simulink model "Traffic_Light_cs"  (R2019b)
settings: Solver=ode5  StartTime=0.0  StopTime=200  FixedStep=1/1000  RelTol=1e-3
PreLoadFcn:
  | mbxruntime.callbacks.PreLoadFcn(bdroot);
PostLoadFcn:
  | mbxruntime.callbacks.PostLoadFcn(bdroot);
InitFcn:
  | mbxruntime.callbacks.InitFcn(bdroot);
StartFcn:
  | mbxruntime.callbacks.StartFcn(bdroot);
StopFcn:
  | mbxruntime.callbacks.StopFcn(bdroot);
model workspace (MAT data in the model file):
  mbox_table : object (value not decoded)
  model_closed = 0
  sim_status = 0
values from neighbouring files (symbols this model uses):
  load_x1 = [-876.8956 -876.745665143 -876.595730285 -876.445795428 -876.29586057 -876.145925713 -875.995990855 -875.846055998 -875.69612114 -875.546186283 -875.396251425 -875.246316568 ... (5741 elements, 5741x1)]    [Data_ckx.mat]    (also in Load.mat)
  load_y1 = [537.3585 537.354079761 537.349659522 537.345239282 537.340819043 537.336398804 537.331978565 537.327558325 537.323138086 537.318717847 537.314297608 537.309877368 ... (5741 elements, 5741x1)]    [Data_ckx.mat]    (also in Load.mat)
  load_z1 = [0 0 0 0 0 0 0 0 0 0 0 0 ... (5741 elements, 5741x1)]    [Data_ckx.mat]    (also in Load.mat)
  q_pass = [0 0 0 37.0489514481 49.8894252687 51.0913174965 61.791576133 65.4762304223 75.669686677 80.4628164105 88.6197377629 94.2384891559 ... (437675 elements, 87535x5)]    [Data_ckx.mat]
  q_stop = [0 0 0 15.0544571491 15.7911831418 16.0935138936 18.6666396431 19.4721381181 21.7098800606 22.5642135149 25.0883481215 26.1253405703 ... (437675 elements, 87535x5)]    [Data_ckx.mat]
  s = roadinf.s    [Constraint_T_V.m]    (also in Light_Distinguish_old.m = 75:-0.7:75-84*0.7)
undefined symbols (not defined in the file or in its folder): InitImageOutputDir, mbxruntime, sigbuilder_block, tabledata
libraries: simulink x10, PreScanSimulinkLibrary x8, simulink_extras x4, autolibshared x1, fuzblock x1
(part 4 of 5)

== system Traffic_Light_cs/CAR_Main/Decision/Function-Call Subsystem/Subsystem ==
  Dis : Inport
  "CameraSensor " : Inport  Port=2
  traffic_state : Inport  Port=3
  TrafficLight_ID_Main : Inport  Port=4
  function : TriggerPort  TriggerType=function-call  VariantControl=Variant
  Bus Selector1 : BusSelector  OutputSignals=ID1,ID2,ID3
  CameraSensor_0919_100_CM_Demux : Subsystem  Tag=demux/Camera/Color  Commented=on  mask{SensorName=CameraSensor_0919_100, hres=1920, vres=1800}
      mask prompts: SensorName "Sensor Name"; hres "Horizontal Resolution"; vres "Vertical Resolution"
      mask Help: eval('openHelp(457)')
      mask Display:
      | fprintf('MONO CAMERA:\n Color\n %s \n %d x %d px',SensorName,hres,vres)
      | port_label('output',1,'R')
      | port_label('output',2,'G')
      | port_label('output',3,'B')
  Constant : Constant  Commented=on  Value=14
  Delay : Stateflow chart  TreatAsAtomicUnit=on
  From : From  Commented=on  GotoTag=R_Ori
  From1 : From  Commented=on  GotoTag=G_Ori
  From2 : From  Commented=on  GotoTag=B_Ori
  Goto : Goto  Commented=on  GotoTag=R_Ori
  Goto1 : Goto  Commented=on  GotoTag=G_Ori
  Goto2 : Goto  Commented=on  GotoTag=B_Ori
  MATLAB Function : MATLAB Function  Commented=on  TreatAsAtomicUnit=on
  MATLAB Function1 : MATLAB Function  TreatAsAtomicUnit=on
  Multiport Switch1 : MultiPortSwitch  DiagnosticForDefault=None
  Product : Product  Commented=on
  Sqrt : Sqrt  Commented=on  SaturateOnIntegerOverflow=on
  Sum : Sum  Commented=on  Inputs=|-+
  Light_State_0919_100 : Outport  VectorParamsAs1DForOutWhenUnconnected=off
  wires:
  Delay/1(Light_State_End) -> Light_State_0919_100/1
  Sqrt/1 -> MATLAB Function/1(Dis)
  Sum/1 -> Sqrt/1
  Constant/1 -> Sum/1
  Product/1 -> Sum/2
  Dis/1 -> MATLAB Function1/1(u), Product/2, Product/1
  From2/1 -> MATLAB Function/4(B_Ori)
  CameraSensor_0919_100_CM_Demux/3(B) -> Goto2/1
  MATLAB Function/1(Light_State) -> ?  "Light_State_0919_100"
  CameraSensor_0919_100_CM_Demux/2(G) -> Goto1/1
  CameraSensor_0919_100_CM_Demux/1(R) -> Goto/1
  "CameraSensor "/1 -> CameraSensor_0919_100_CM_Demux/1(In1)
  From1/1 -> MATLAB Function/3(G_Ori)
  From/1 -> MATLAB Function/2(R_Ori)
  Multiport Switch1/1 -> MATLAB Function1/2(data)
  traffic_state/1 -> Bus Selector1/1
  Bus Selector1/1 -> Multiport Switch1/2  "<ID1>"
  Bus Selector1/2 -> Multiport Switch1/3  "<ID2>"
  Bus Selector1/3 -> Multiport Switch1/4  "<ID3>"
  TrafficLight_ID_Main/1 -> Multiport Switch1/1
  MATLAB Function1/1(y) -> Delay/1(Light_State_0919_100)

== system Traffic_Light_cs/CAR_Main/Dynamics_Simple/Chassis/Bicycle_model_[XYZ] ==
  DeltaWheel_[rad] : Inport
  zFront_[m]_dzFront_[ms-1] : Inport  Port=2  PortDimensions=2
  zRear_[m]_dzRear_[ms-1] : Inport  Port=3  PortDimensions=2
  |vx|_[ms-1] : Inport  Port=4
  Fy_rear_[N] : Inport  Port=5
  Fy_front_[N] : Inport  Port=6
  Demux : Demux  Outputs=2
  Demux1 : Demux  Outputs=2
  Fyi --> Fy / Mz : Subsystem
  Y & Yaw_Motion : Subsystem
  "Z, Pitch_Motion & Roll_Motion" : Subsystem
  |vx|_[ms-1]1 : Outport  VectorParamsAs1DForOutWhenUnconnected=off
  vy_[ms-1] : Outport  Port=2  VectorParamsAs1DForOutWhenUnconnected=off
  vz_[ms-1] : Outport  Port=3  VectorParamsAs1DForOutWhenUnconnected=off
  RollAngle_[rad] : Outport  Port=4  VectorParamsAs1DForOutWhenUnconnected=off
  RollRate_[rads-1] : Outport  Port=5  VectorParamsAs1DForOutWhenUnconnected=off
  YawAngle_[rads-1] : Outport  Port=6  VectorParamsAs1DForOutWhenUnconnected=off
  PitchAngle_[rad] : Outport  Port=7  VectorParamsAs1DForOutWhenUnconnected=off
  YawAngle_[rad] : Outport  Port=8  VectorParamsAs1DForOutWhenUnconnected=off
  ay_[ms-2] : Outport  Port=9  VectorParamsAs1DForOutWhenUnconnected=off
  wires:
  "Z, Pitch_Motion & Roll_Motion"/1(pitchAngle_[rad]) -> PitchAngle_[rad]/1  "PitchAngle_[rad]"
  Y & Yaw_Motion/4(dYawAngle_[rads-1]) -> [dYaw], YawAngle_[rads-1]/1  "dYawAngle_[rads-1]"
  [vx] -> "Z, Pitch_Motion & Roll_Motion"/1(vx)
  [dYaw] -> "Z, Pitch_Motion & Roll_Motion"/2(dYaw)
  "Z, Pitch_Motion & Roll_Motion"/4(RollRate_[rads-1]) -> RollRate_[rads-1]/1  "RollRate_[rads-1]"
  "Z, Pitch_Motion & Roll_Motion"/3(RollAngle_[rad]) -> RollAngle_[rad]/1  "RollAngle_[rad]"
  [ay] -> "Z, Pitch_Motion & Roll_Motion"/4(ay)
  Y & Yaw_Motion/3(ay_[ms-2]) -> ay_[ms-2]/1, [ay]  "ay_[ms-2]"
  |vx|_[ms-1]/1 -> Y & Yaw_Motion/1(|vx|_[ms-1])
  Fy_rear_[N]/1 -> Fyi --> Fy / Mz/3(Fy_r_[N])
  Fy_front_[N]/1 -> Fyi --> Fy / Mz/2(Fy_f_[N])
  DeltaWheel_[rad]/1 -> Fyi --> Fy / Mz/1(DeltaWheel_[rad])
  "Z, Pitch_Motion & Roll_Motion"/2(vz_[ms-1]) -> vz_[ms-1]/1  "vz_[ms-1]"
  zFront_[m]_dzFront_[ms-1]/1 -> Demux/1
  zRear_[m]_dzRear_[ms-1]/1 -> Demux1/1
  Demux1/2 -> "Z, Pitch_Motion & Roll_Motion"/8(dzRear_[ms-1])
  Demux1/1 -> "Z, Pitch_Motion & Roll_Motion"/7(zRear_[m])
  Demux/2 -> "Z, Pitch_Motion & Roll_Motion"/6(dzFront_[ms-1])
  Demux/1 -> "Z, Pitch_Motion & Roll_Motion"/5(zFront_[m])
  [ax] -> "Z, Pitch_Motion & Roll_Motion"/3(ax)
  Y & Yaw_Motion/5(YawAngle_[rad]) -> YawAngle_[rad]/1  "YawAngle_[rad]"
  Y & Yaw_Motion/2(vy_[ms-1]) -> vy_[ms-1]/1  "vy_[ms-1]"
  Y & Yaw_Motion/1(|vx|_[ms-1]1) -> |vx|_[ms-1]1/1  "|vx|_[ms-1]"
  Fyi --> Fy / Mz/2(Mz_[Nm]) -> Y & Yaw_Motion/3(Mz_[Nm])  "Mz_[Nm]"
  Fyi --> Fy / Mz/1(Fy_[N]) -> Y & Yaw_Motion/2(Fy_[N])  "Fy_[N]"

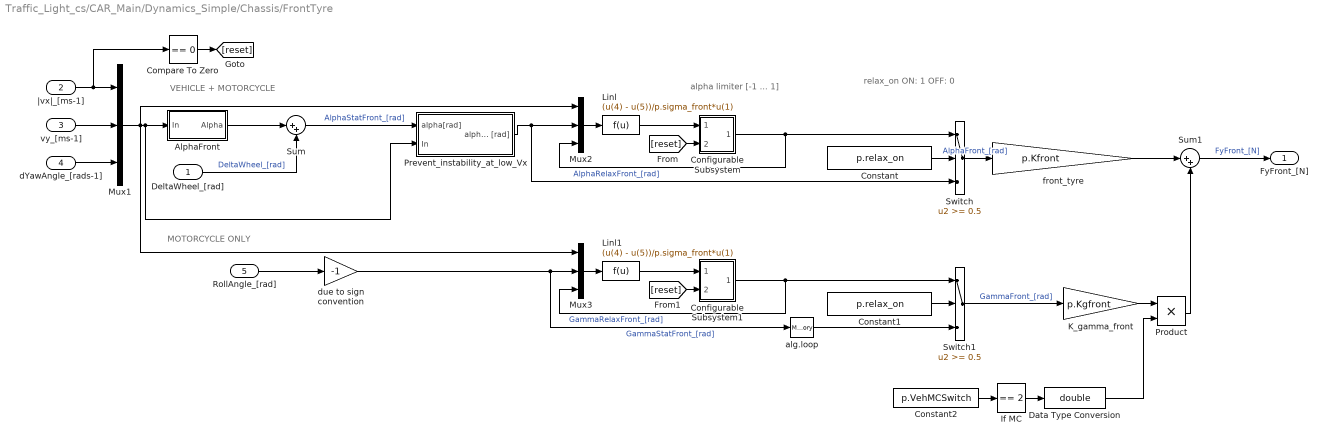
== system Traffic_Light_cs/CAR_Main/Dynamics_Simple/Chassis/FrontTyre ==
  note: VEHICLE + MOTORCYCLE
  note: MOTORCYCLE ONLY
  note: relax_on
      | ON: 1
      | OFF: 0
  note: alpha limiter
      | [-1 ... 1]
  DeltaWheel_[rad] : Inport
  |vx|_[ms-1] : Inport  Port=2
  vy_[ms-1] : Inport  Port=3
  dYawAngle_[rads-1] : Inport  Port=4
  RollAngle_[rad] : Inport  Port=5
  AlphaFront : Subsystem
  Compare To Zero : simulink/Logic and Bit Operations/Compare To Zero  relop===  OutDataTypeStr=boolean  ZeroCross=off
  Configurable Subsystem : Subsystem  BlockChoice=Integrator  mask{ComputationMode=ComputationMode}
      mask prompts: ComputationMode "Computation mode:"
      mask init:
      | SetComputationMode(gcb,ComputationMode);
      settings: AttributesFormatString=%<BlockChoice>  OpenFcn=BringToFront(gcb);  MemberBlocks=Discrete-Time Integrator,Integrator
      settings: TemplateBlock=|
      | PreScanSimulinkLibrary/Configurable Subsystems/integral with reset and limits
      | for slip angle/Configurable
      | Subsystem
  Configurable Subsystem1 : Subsystem  BlockChoice=Integrator  mask{ComputationMode=ComputationMode}
      mask prompts: ComputationMode "Computation mode:"
      mask init:
      | SetComputationMode(gcb,ComputationMode);
      settings: AttributesFormatString=%<BlockChoice>  OpenFcn=BringToFront(gcb);  MemberBlocks=Discrete-Time Integrator,Integrator
      settings: TemplateBlock=|
      | PreScanSimulinkLibrary/Configurable Subsystems/integral with reset/Configurable
      | Subsystem
  Constant : Constant  Value=p.relax_on
  Constant1 : Constant  Value=p.relax_on
  Constant2 : Constant  Value=p.VehMCSwitch
  Data Type Conversion : DataTypeConversion  OutDataTypeStr=double
  If MC : simulink/Logic and Bit Operations/Compare To Constant  relop===  const=2  OutDataTypeStr=uint8  ZeroCross=off
  K_gamma_front : Gain  Gain=p.Kgfront
  Linl : Fcn  Expr=(u(4) - u(5))/p.sigma_front*u(1)
  Linl1 : Fcn  Expr=(u(4) - u(5))/p.sigma_front*u(1)
  Mux1 : Mux  Inputs=3
  Mux2 : Mux  Inputs={3,1,1}
  Mux3 : Mux  Inputs={3,1,1}
  Prevent_instability_at_low_Vx : Subsystem
  Product : Product  RndMeth=Zero
  Sum : Sum  Inputs=|++  SaturateOnIntegerOverflow=on  InputSameDT=on  OutDataTypeStr=Inherit: Same as first input
  Sum1 : Sum  Inputs=|++
  Switch : Switch  Threshold=0.5  SaturateOnIntegerOverflow=on  InputSameDT=on
  Switch1 : Switch  Threshold=0.5  SaturateOnIntegerOverflow=on  InputSameDT=on
  alg.loop : Memory
  due to sign convention : Gain  Gain=-1  SaturateOnIntegerOverflow=on  OutDataTypeStr=Inherit: Same as input  ParamDataTypeStr=Inherit: Same as input
  front_tyre : Gain  Gain=p.Kfront
  FyFront_[N] : Outport  VectorParamsAs1DForOutWhenUnconnected=off
  wires:
  Switch1/1 -> K_gamma_front/1  "GammaFront_[rad]"
  DeltaWheel_[rad]/1 -> Sum/2  "DeltaWheel_[rad]"
  [reset] -> Configurable Subsystem1/2(In2)
  [reset] -> Configurable Subsystem/2(In2)
  Compare To Zero/1 -> [reset]
  Data Type Conversion/1 -> Product/2
  Product/1 -> Sum1/2
  K_gamma_front/1 -> Product/1
  If MC/1 -> Data Type Conversion/1
  Constant2/1 -> If MC/1
  front_tyre/1 -> Sum1/1
  RollAngle_[rad]/1 -> due to sign convention/1
  due to sign convention/1 -> Mux3/2, alg.loop/1  "GammaStatFront_[rad]"
  Constant1/1 -> Switch1/2
  Mux3/1 -> Linl1/1
  Linl1/1 -> Configurable Subsystem1/1(In1)
  Configurable Subsystem1/1(Out1) -> Switch1/1, Mux3/3  "GammaRelaxFront_[rad]"
  alg.loop/1 -> Switch1/3
  dYawAngle_[rads-1]/1 -> Mux1/3
  vy_[ms-1]/1 -> Mux1/2
  |vx|_[ms-1]/1 -> Compare To Zero/1, Mux1/1
  Mux1/1 -> Mux3/1, Mux2/1, AlphaFront/1(In), Prevent_instability_at_low_Vx/2(In)
  AlphaFront/1(Alpha) -> Sum/1
  Configurable Subsystem/1(Out1) -> Switch/1, Mux2/3  "AlphaRelaxFront_[rad]"
  Linl/1 -> Configurable Subsystem/1(In1)
  Mux2/1 -> Linl/1
  Sum1/1 -> FyFront_[N]/1  "FyFront_[N]"
  Constant/1 -> Switch/2
  Switch/1 -> front_tyre/1  "AlphaFront_[rad]"
  Sum/1 -> Prevent_instability_at_low_Vx/1(alpha[rad])  "AlphaStatFront_[rad]"
  Prevent_instability_at_low_Vx/1(alpha [rad]) -> Switch/3, Mux2/2

== system Traffic_Light_cs/CAR_Main/Dynamics_Simple/Chassis/MuxDynState ==
  note: AnglesVEHICLE
      | wrtGLOB
  note: mode: Dynamics
      | VelVEHICLE
      | wrt VEH
  note: The position inputs are computed by the
      | integrated velocity.
  vx [ms-1] : Inport
  vy [ms-1] : Inport  Port=2
  vz [ms-1] : Inport  Port=3
  R [rad] : Inport  Port=4
  P [rad] : Inport  Port=5
  Y [rad] : Inport  Port=6
  Configurable Subsystem1 : Subsystem  BlockChoice=Integrator  mask{ComputationMode=ComputationMode}
      mask prompts: ComputationMode "Computation mode:"
      mask init:
      | SetComputationMode(gcb,ComputationMode);
      settings: AttributesFormatString=%<BlockChoice>  OpenFcn=BringToFront(gcb);  MemberBlocks=Discrete-Time Integrator,Integrator
      settings: TemplateBlock=|
      | PreScanSimulinkLibrary/Configurable Subsystems/integral/Configurable
      | Subsystem1
  Ground : Ground
  Ground1 : Ground
  Mux : Mux  Inputs=[3 3 3]
  Mux1 : Mux  Inputs=3
  Mux2 : Mux  Inputs=3
  Transformation_BODY2GLOBAL : Subsystem
  mux3 : Mux  Inputs=3
  State : Outport  VectorParamsAs1DForOutWhenUnconnected=off
  wires:
  Configurable Subsystem1/1(Out1) -> Mux/1  "PosVEH wrt  GLOB"
  Mux1/1 -> Transformation_BODY2GLOBAL/1(Vvector_BODY_[m/s])
  Mux/1 -> State/1
  Ground/1 -> mux3/1  "roll"
  mux3/1 -> Transformation_BODY2GLOBAL/2(angles_BODYwrtGLOB_[rad])
  Transformation_BODY2GLOBAL/1(Vvector_GLOBAL_[m/s]) -> Mux/2, Configurable Subsystem1/1(In1)  "VelVEH wrt  GLOB"
  Mux2/1 -> Mux/3
  vx [ms-1]/1 -> Mux1/1
  vy [ms-1]/1 -> Mux1/2
  vz [ms-1]/1 -> Mux1/3
  R [rad]/1 -> Mux2/1
  P [rad]/1 -> Mux2/2
  Y [rad]/1 -> mux3/3, Mux2/3  "yaw"
  Ground1/1 -> mux3/2  "pitch"

== system Traffic_Light_cs/CAR_Main/Dynamics_Simple/Chassis/Power Assisted Steering ==
  note: Reverse steering direction for negative velocities
  note: VEHICLE
  note: MOTORCYCLE
  Vx_[ms-1] : Inport
  Delta_in_[deg] : Inport  Port=2
  Constant : Constant
  Constant1 : Constant  Value=p.VehMCSwitch
  Lookup Table : Lookup  InputValues=[0 35 45 100]  Table=[1 1 0.2 0.2]
  Multiport Switch : MultiPortSwitch  Inputs=2
  Product : Product  Inputs=3  RndMeth=Zero
  Sign : Signum
  Delta_out_[deg] : Outport  VectorParamsAs1DForOutWhenUnconnected=off
  wires:
  Sign/1 -> Product/1
  Product/1 -> Delta_out_[deg]/1
  Multiport Switch/1 -> Product/2
  Lookup Table/1 -> Multiport Switch/2
  Constant/1 -> Multiport Switch/3
  Constant1/1 -> Multiport Switch/1
  Delta_in_[deg]/1 -> Product/3
  Vx_[ms-1]/1 -> Sign/1, Lookup Table/1

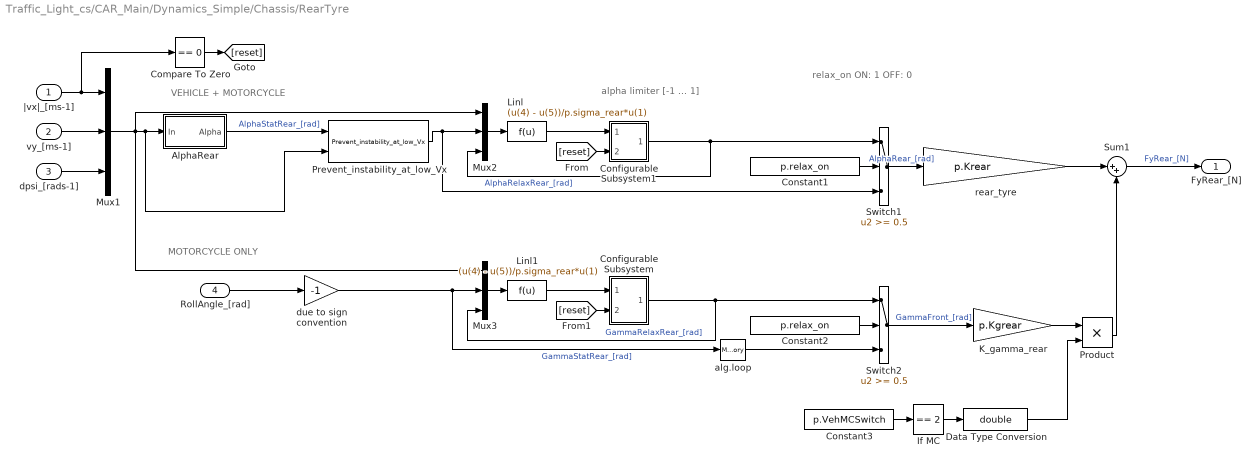
== system Traffic_Light_cs/CAR_Main/Dynamics_Simple/Chassis/RearTyre ==
  note: VEHICLE + MOTORCYCLE
  note: MOTORCYCLE ONLY
  note: relax_on
      | ON: 1
      | OFF: 0
  note: alpha limiter
      | [-1 ... 1]
  |vx|_[ms-1] : Inport
  vy_[ms-1] : Inport  Port=2
  dpsi_[rads-1] : Inport  Port=3
  RollAngle_[rad] : Inport  Port=4
  AlphaRear : Subsystem
  Compare To Zero : simulink/Logic and Bit Operations/Compare To Zero  relop===  OutDataTypeStr=boolean  ZeroCross=off
  Configurable Subsystem : Subsystem  BlockChoice=Integrator  mask{ComputationMode=ComputationMode}
      mask prompts: ComputationMode "Computation mode:"
      mask init:
      | SetComputationMode(gcb,ComputationMode);
      settings: AttributesFormatString=%<BlockChoice>  OpenFcn=BringToFront(gcb);  MemberBlocks=Discrete-Time Integrator,Integrator
      settings: TemplateBlock=|
      | PreScanSimulinkLibrary/Configurable Subsystems/integral with reset/Configurable
      | Subsystem
  Configurable Subsystem1 : Subsystem  BlockChoice=Integrator  mask{ComputationMode=ComputationMode}
      mask prompts: ComputationMode "Computation mode:"
      mask init:
      | SetComputationMode(gcb,ComputationMode);
      settings: AttributesFormatString=%<BlockChoice>  OpenFcn=BringToFront(gcb);  MemberBlocks=Discrete-Time Integrator,Integrator
      settings: TemplateBlock=|
      | PreScanSimulinkLibrary/Configurable Subsystems/integral with reset and limits
      | for slip angle/Configurable
      | Subsystem
  Constant1 : Constant  Value=p.relax_on
  Constant2 : Constant  Value=p.relax_on
  Constant3 : Constant  Value=p.VehMCSwitch
  Data Type Conversion : DataTypeConversion  OutDataTypeStr=double
  If MC : simulink/Logic and Bit Operations/Compare To Constant  relop===  const=2  OutDataTypeStr=uint8  ZeroCross=off
  K_gamma_rear : Gain  Gain=p.Kgrear
  Linl : Fcn  Expr=(u(4) - u(5))/p.sigma_rear*u(1)
  Linl1 : Fcn  Expr=(u(4) - u(5))/p.sigma_rear*u(1)
  Mux1 : Mux  Inputs=3
  Mux2 : Mux  Inputs={3,1,1}
  Mux3 : Mux  Inputs={3,1,1}
  Prevent_instability_at_low_Vx : PreScanSimulinkLibrary/Simple_Vehicle_Dynamics/Chassis/FrontTyre/Prevent_instability_at_low_Vx  SystemSampleTime=-1  Latency=0  AutoFrameSizeCalculation=off
  Product : Product  RndMeth=Zero
  Sum1 : Sum  Inputs=|++
  Switch1 : Switch  Threshold=0.5  SaturateOnIntegerOverflow=on  InputSameDT=on
  Switch2 : Switch  Threshold=0.5  SaturateOnIntegerOverflow=on  InputSameDT=on
  alg.loop : Memory
  due to sign convention : Gain  Gain=-1  SaturateOnIntegerOverflow=on  OutDataTypeStr=Inherit: Same as input  ParamDataTypeStr=Inherit: Same as input
  rear_tyre : Gain  Gain=p.Krear
  FyRear_[N] : Outport  VectorParamsAs1DForOutWhenUnconnected=off
  wires:
  Switch2/1 -> K_gamma_rear/1  "GammaFront_[rad]"
  [reset] -> Configurable Subsystem/2(In2)
  [reset] -> Configurable Subsystem1/2(In2)
  Compare To Zero/1 -> [reset]
  rear_tyre/1 -> Sum1/1
  K_gamma_rear/1 -> Product/1
  Data Type Conversion/1 -> Product/2
  Product/1 -> Sum1/2
  If MC/1 -> Data Type Conversion/1
  Constant3/1 -> If MC/1
  RollAngle_[rad]/1 -> due to sign convention/1
  due to sign convention/1 -> Mux3/2, alg.loop/1  "GammaStatRear_[rad]"
  Constant2/1 -> Switch2/2
  Mux3/1 -> Linl1/1
  Linl1/1 -> Configurable Subsystem/1(In1)
  Configurable Subsystem/1(Out1) -> Switch2/1, Mux3/3  "GammaRelaxRear_[rad]"
  alg.loop/1 -> Switch2/3
  dpsi_[rads-1]/1 -> Mux1/3
  vy_[ms-1]/1 -> Mux1/2
  |vx|_[ms-1]/1 -> Compare To Zero/1, Mux1/1
  Mux1/1 -> Mux3/1, Mux2/1, Prevent_instability_at_low_Vx/2, AlphaRear/1(In)
  Configurable Subsystem1/1(Out1) -> Switch1/1, Mux2/3  "AlphaRelaxRear_[rad]"
  Linl/1 -> Configurable Subsystem1/1(In1)
  Mux2/1 -> Linl/1
  Sum1/1 -> FyRear_[N]/1  "FyRear_[N]"
  Constant1/1 -> Switch1/2
  Switch1/1 -> rear_tyre/1  "AlphaRear_[rad]"
  AlphaRear/1(Alpha) -> Prevent_instability_at_low_Vx/1  "AlphaStatRear_[rad]"
  Prevent_instability_at_low_Vx/1 -> Mux2/2, Switch1/3

== system Traffic_Light_cs/CAR_Main/SELF_Demux/compas converter/cart2compas ==
  Angle [deg] : Inport
  Constant : Constant  Value=90
  Constant1 : Constant  Value=360
  Gain : Gain  Gain=1/360
  Gain1 : Gain  Gain=360
  Gain2 : Gain  Gain=-1
  Rounding Function : Rounding
  Sum : Sum  Inputs=|-+
  Sum1 : Sum  Inputs=-+|
  Sum2 : Sum  Inputs=++|
  heading [deg] : Outport
  wires:
  Gain/1 -> Rounding Function/1
  Rounding Function/1 -> Gain1/1
  Gain1/1 -> Sum/1
  Angle [deg]/1 -> Sum1/2
  Sum/1 -> Gain2/1
  Sum1/1 -> Gain/1, Sum/2
  Constant/1 -> Sum1/1
  Gain2/1 -> Sum2/2
  Constant1/1 -> Sum2/1
  Sum2/1 -> heading [deg]/1

== system Traffic_Light_cs/CAR_Main/pre/Subsystem/Signal Builder ==
  Demux : Demux  Tag=STV Demux  Outputs=6
  FromWs : FromWorkspace  Tag=STV FromWs  VariableName=tuvar  SampleTime=0
      SigBuilderData=|
      | common.afterFinalStr = 'Extrapolate'
      | common.sampleTime = 0
      | dataSet.timeRange = [0 200]
      | dataSet.name = 'Traffic Light GPS Information'
      | sbobj.Groups.Name = 'Traffic Light GPS Information'
      | sbobj.Groups.Signals(1).Name = 'ID==1,X'
      | sbobj.Groups.Signals(1).XData = [0 200]
      | sbobj.Groups.Signals(1).YData = [-610.5 -610.5]
      | sbobj.Groups.Signals(2).Name = 'ID==1,Y'
      | sbobj.Groups.Signals(2).XData = [0 200]
      | sbobj.Groups.Signals(2).YData = [362.27 362.27]
      | sbobj.Groups.Signals(3).Name = 'ID==2,X'
      | sbobj.Groups.Signals(3).XData = [0 200]
      | sbobj.Groups.Signals(3).YData = [-639.42 -639.42]
      | sbobj.Groups.Signals(4).Name = 'ID==2,Y'
      | sbobj.Groups.Signals(4).XData = [0 200]
      | sbobj.Groups.Signals(4).YData = [295.94 295.94]
      | sbobj.Groups.Signals(5).Name = 'ID==3,X'
      | sbobj.Groups.Signals(5).XData = [0 200]
      | sbobj.Groups.Signals(5).YData = [-718.98 -718.98]
      | sbobj.Groups.Signals(6).Name = 'ID==3,Y'
      | sbobj.Groups.Signals(6).XData = [0 200]
      | sbobj.Groups.Signals(6).YData = [201.74 201.74]
      | sbobj.Groups.TimeRange = [0 200]
  ID==1,X : Outport  Tag=STV Outport
  ID==1,Y : Outport  Tag=STV Outport  Port=2  VectorParamsAs1DForOutWhenUnconnected=off
  ID==2,X : Outport  Tag=STV Outport  Port=3  VectorParamsAs1DForOutWhenUnconnected=off
  ID==2,Y : Outport  Tag=STV Outport  Port=4  VectorParamsAs1DForOutWhenUnconnected=off
  ID==3,X : Outport  Tag=STV Outport  Port=5  VectorParamsAs1DForOutWhenUnconnected=off
  ID==3,Y : Outport  Tag=STV Outport  Port=6  VectorParamsAs1DForOutWhenUnconnected=off
  wires:
  Demux/6 -> ID==3,Y/1
  Demux/5 -> ID==3,X/1
  Demux/4 -> ID==2,Y/1
  Demux/3 -> ID==2,X/1
  Demux/2 -> ID==1,Y/1
  Demux/1 -> ID==1,X/1
  FromWs/1 -> Demux/1

== system Traffic_Light_cs/CAR_Ahead/Decision/Function-Call Subsystem/Subsystem/CameraSensor_0919_100_CM_Demux ==
  In1 : Inport
  Selector : Selector  NumberOfDimensions=2  InputPortWidth=3  IndexOptions=Index vector (dialog),Index vector (dialog)  Indices=-1,1:hres  OutputSizes=1,1
  Selector1 : Selector  NumberOfDimensions=2  InputPortWidth=3  IndexOptions=Index vector (dialog),Index vector (dialog)  Indices=-1,hres+1:hres*2  OutputSizes=1,1
  Selector2 : Selector  NumberOfDimensions=2  InputPortWidth=3  IndexOptions=Index vector (dialog),Index vector (dialog)  Indices=-1,hres*2+1:hres*3  OutputSizes=1,1
  R : Outport  VectorParamsAs1DForOutWhenUnconnected=off
  G : Outport  Port=2  VectorParamsAs1DForOutWhenUnconnected=off
  B : Outport  Port=3  VectorParamsAs1DForOutWhenUnconnected=off
  wires:
  Selector2/1 -> B/1
  Selector1/1 -> G/1
  Selector/1 -> R/1
  In1/1 -> Selector2/1, Selector/1, Selector1/1

== system Traffic_Light_cs/CAR_Ahead/Trajectories/Traj2State1/Traj2State2/MuxState ==
  x [m] : Inport
  y [m] : Inport  Port=2
  z [m] : Inport  Port=3
  dx [m/s] : Inport  Port=4
  dy [m/s] : Inport  Port=5
  dz [m/s] : Inport  Port=6
  R [rad] : Inport  Port=7
  P [rad] : Inport  Port=8
  Y [rad] : Inport  Port=9
  Mux : Mux  Inputs=9
  state : Outport
  wires:
  z [m]/1 -> Mux/3
  y [m]/1 -> Mux/2
  x [m]/1 -> Mux/1
  Y [rad]/1 -> Mux/9
  P [rad]/1 -> Mux/8
  R [rad]/1 -> Mux/7
  dz [m/s]/1 -> Mux/6
  dy [m/s]/1 -> Mux/5
  dx [m/s]/1 -> Mux/4
  Mux/1 -> state/1

== system Traffic_Light_cs/CAR_Ahead/Trajectories/Traj2State1/Traj2State2/Traj2MuxState_Ext ==
  Traj : Inport
  Terminator{1..9} (9 alike) : Terminator
  demux : Subsystem
  x [m] : Outport
  y [m] : Outport  Port=2
  z [m] : Outport  Port=3
  dx [m/s] : Outport  Port=4
  dy [m/s] : Outport  Port=5
  dz [m/s] : Outport  Port=6
  R [rad] : Outport  Port=7
  P [rad] : Outport  Port=8
  Y [rad] : Outport  Port=9
  wires:
  demux/9(Y) -> Y [rad]/1
  demux/7(R) -> R [rad]/1
  demux/5(vely) -> dy [m/s]/1
  demux/4(velx) -> dx [m/s]/1
  demux/10(velR) -> Terminator4/1
  demux/11(velP) -> Terminator5/1
  demux/12(velY) -> Terminator1/1
  demux/13(accx) -> Terminator8/1
  demux/14(accy) -> Terminator9/1
  demux/15(accz) -> Terminator7/1
  demux/18(accY) -> Terminator2/1
  demux/16(accR) -> Terminator3/1
  demux/17(accP) -> Terminator6/1
  demux/3(z) -> z [m]/1
  Traj/1 -> demux/1(traj)
  demux/6(velz) -> dz [m/s]/1
  demux/1(x) -> x [m]/1
  demux/2(y) -> y [m]/1
  demux/8(P) -> P [rad]/1

== system Traffic_Light_cs/CAR_Main/Decision/Function-Call Subsystem/Subsystem/CameraSensor_0919_100_CM_Demux ==
  In1 : Inport
  Selector : Selector  NumberOfDimensions=2  InputPortWidth=3  IndexOptions=Index vector (dialog),Index vector (dialog)  Indices=-1,1:hres  OutputSizes=1,1
  Selector1 : Selector  NumberOfDimensions=2  InputPortWidth=3  IndexOptions=Index vector (dialog),Index vector (dialog)  Indices=-1,hres+1:hres*2  OutputSizes=1,1
  Selector2 : Selector  NumberOfDimensions=2  InputPortWidth=3  IndexOptions=Index vector (dialog),Index vector (dialog)  Indices=-1,hres*2+1:hres*3  OutputSizes=1,1
  R : Outport  VectorParamsAs1DForOutWhenUnconnected=off
  G : Outport  Port=2  VectorParamsAs1DForOutWhenUnconnected=off
  B : Outport  Port=3  VectorParamsAs1DForOutWhenUnconnected=off
  wires:
  Selector2/1 -> B/1
  Selector1/1 -> G/1
  Selector/1 -> R/1
  In1/1 -> Selector2/1, Selector/1, Selector1/1

== system Traffic_Light_cs/CAR_Main/Dynamics_Simple/Chassis/Bicycle_model_[XYZ]/Fyi --> Fy // Mz ==
  DeltaWheel_[rad] : Inport
  Fy_f_[N] : Inport  Port=2
  Fy_r_[N] : Inport  Port=3
  Fy : Fcn  Expr=u(2)*cos(u(1)) + u(3)
  Mux1 : Mux  Inputs=3
  Mz : Fcn  Expr=u(2)*p.a*cos(u(1)) - u(3)*p.b
  Fy_[N] : Outport  InitialOutput=0  VectorParamsAs1DForOutWhenUnconnected=off
  Mz_[Nm] : Outport  Port=2  InitialOutput=0  VectorParamsAs1DForOutWhenUnconnected=off
  wires:
  Fy_r_[N]/1 -> Mux1/3
  Fy_f_[N]/1 -> Mux1/2
  Mux1/1 -> Fy/1, Mz/1
  Fy/1 -> Fy_[N]/1
  Mz/1 -> Mz_[Nm]/1
  DeltaWheel_[rad]/1 -> Mux1/1  "DeltaWheel_[rad]"

== system Traffic_Light_cs/CAR_Main/Dynamics_Simple/Chassis/Bicycle_model_[XYZ]/Y & Yaw_Motion ==
  |vx|_[ms-1] : Inport
  Fy_[N] : Inport  Port=2
  Mz_[Nm] : Inport  Port=3
  Compare To Zero : simulink/Logic and Bit Operations/Compare To Zero  relop===  OutDataTypeStr=boolean  ZeroCross=off
  Configurable Subsystem : Subsystem  BlockChoice=Integrator  mask{ComputationMode=ComputationMode}
      mask prompts: ComputationMode "Computation mode:"
      mask init:
      | SetComputationMode(gcb,ComputationMode);
      settings: AttributesFormatString=%<BlockChoice>  OpenFcn=BringToFront(gcb);  MemberBlocks=Discrete-Time Integrator,Integrator
      settings: TemplateBlock=|
      | PreScanSimulinkLibrary/Configurable Subsystems/integral with reset/Configurable
      | Subsystem
  Configurable Subsystem1 : Subsystem  BlockChoice=Integrator  mask{ComputationMode=ComputationMode}
      link override Discrete-Time Integrator: IntegratorMethod=Integration: Backward Euler
      mask prompts: ComputationMode "Computation mode:"
      mask init:
      | SetComputationMode(gcb,ComputationMode);
      settings: AttributesFormatString=%<BlockChoice>  OpenFcn=BringToFront(gcb);  MemberBlocks=Discrete-Time Integrator,Integrator
      settings: TemplateBlock=|
      | PreScanSimulinkLibrary/Configurable Subsystems/integral/Configurable
      | Subsystem1
  Configurable Subsystem2 : Subsystem  BlockChoice=Integrator  mask{ComputationMode=ComputationMode}
      mask prompts: ComputationMode "Computation mode:"
      mask init:
      | SetComputationMode(gcb,ComputationMode);
      settings: AttributesFormatString=%<BlockChoice>  OpenFcn=BringToFront(gcb);  MemberBlocks=Discrete-Time Integrator,Integrator
      settings: TemplateBlock=|
      | PreScanSimulinkLibrary/Configurable Subsystems/integral with reset/Configurable
      | Subsystem
  Fcn1 : Fcn  Expr=u(1)*u(3)
  Gain : Gain  Gain=1/p.m  SaturateOnIntegerOverflow=on  OutDataTypeStr=Inherit: Same as input  ParamDataTypeStr=Inherit: Same as input
  Gain1 : Gain  Gain=1/p.J_zz  SaturateOnIntegerOverflow=on  OutDataTypeStr=Inherit: Same as input  ParamDataTypeStr=Inherit: Same as input
  Sum1 : Sum  Inputs=-+  SaturateOnIntegerOverflow=on  InputSameDT=on  OutDataTypeStr=Inherit: Same as first input
  mux : Mux  Inputs=3
  |vx|_[ms-1]1 : Outport  InitialOutput=0  VectorParamsAs1DForOutWhenUnconnected=off
  vy_[ms-1] : Outport  Port=2  InitialOutput=0  VectorParamsAs1DForOutWhenUnconnected=off
  ay_[ms-2] : Outport  Port=3  InitialOutput=0  VectorParamsAs1DForOutWhenUnconnected=off
  dYawAngle_[rads-1] : Outport  Port=4  InitialOutput=0  VectorParamsAs1DForOutWhenUnconnected=off
  YawAngle_[rad] : Outport  Port=5  InitialOutput=0  VectorParamsAs1DForOutWhenUnconnected=off
  wires:
  Gain1/1 -> Configurable Subsystem2/1(In1)  "ddYawAngle_[rads-2]"
  Gain/1 -> Sum1/2, ay_[ms-2]/1  "ddy_[ms-2]"
  [reset] -> Configurable Subsystem/2(In2)
  [reset] -> Configurable Subsystem2/2(In2)
  Compare To Zero/1 -> [reset]
  Configurable Subsystem1/1(Out1) -> YawAngle_[rad]/1
  Mz_[Nm]/1 -> Gain1/1  "Mz_[Nm]"
  Fy_[N]/1 -> Gain/1  "Fy_[N]"
  Sum1/1 -> Configurable Subsystem/1(In1)  "dvy_[ms-2]"
  Fcn1/1 -> Sum1/1  "|vx|*dYawAngle_[ms-2]"
  mux/1 -> Fcn1/1  "|vx|_[ms-1]_vy_[ms-1]_dYawAngle_[rads-1]"
  |vx|_[ms-1]/1 -> Compare To Zero/1, |vx|_[ms-1]1/1, mux/1  "|vx|_[ms-1]"
  Configurable Subsystem/1(Out1) -> vy_[ms-1]/1, mux/2  "vy_[ms-1]"
  Configurable Subsystem2/1(Out1) -> dYawAngle_[rads-1]/1, mux/3, Configurable Subsystem1/1(In1)  "dYawAngle_[rads-1]"

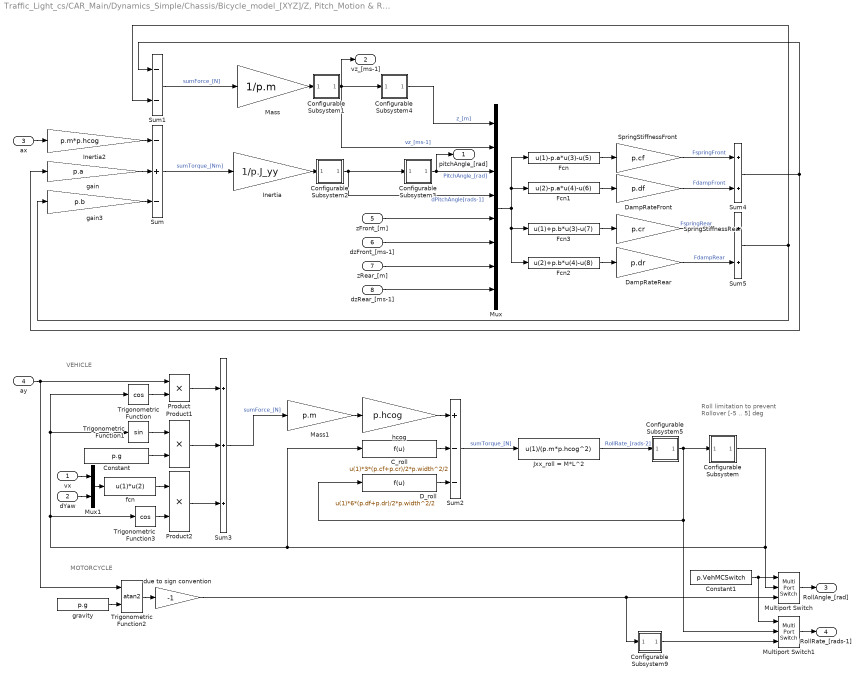
== system Traffic_Light_cs/CAR_Main/Dynamics_Simple/Chassis/Bicycle_model_[XYZ]/Z, Pitch_Motion & Roll_Motion ==
  note: Roll limitation
      | to prevent
      | Rollover
      | [-5 .. 5] deg
  note: VEHICLE
  note: MOTORCYCLE
  vx : Inport
  dYaw : Inport  Port=2
  ax : Inport  Port=3
  ay : Inport  Port=4
  zFront_[m] : Inport  Port=5
  dzFront_[ms-1] : Inport  Port=6
  zRear_[m] : Inport  Port=7
  dzRear_[ms-1] : Inport  Port=8
  C_roll : Fcn  Expr=u(1)*3*(p.cf+p.cr)/2*p.width^2/2
  Configurable Subsystem : Subsystem  BlockChoice=Integrator  mask{ComputationMode=ComputationMode}
      link override Discrete-Time Integrator: UpperSaturationLimit=5*pi/180  LowerSaturationLimit=-5*pi/180
      link override Integrator: UpperSaturationLimit=5*pi/180  LowerSaturationLimit=-5*pi/180
      mask prompts: ComputationMode "Computation mode:"
      mask init:
      | SetComputationMode(gcb,ComputationMode);
      settings: AttributesFormatString=%<BlockChoice>  OpenFcn=BringToFront(gcb);  MemberBlocks=Discrete-Time Integrator,Integrator
      settings: TemplateBlock=|
      | PreScanSimulinkLibrary/Configurable Subsystems/integral with limits
      | for roll motion/Configurable
      | Subsystem
  Configurable Subsystem1 : Subsystem  BlockChoice=Integrator  mask{ComputationMode=ComputationMode}
      mask prompts: ComputationMode "Computation mode:"
      mask init:
      | SetComputationMode(gcb,ComputationMode);
      settings: AttributesFormatString=%<BlockChoice>  OpenFcn=BringToFront(gcb);  MemberBlocks=Discrete-Time Integrator,Integrator
      settings: TemplateBlock=|
      | PreScanSimulinkLibrary/Configurable Subsystems/integral/Configurable
      | Subsystem1
  Configurable Subsystem2 : Subsystem  BlockChoice=Integrator  mask{ComputationMode=ComputationMode}
      mask prompts: ComputationMode "Computation mode:"
      mask init:
      | SetComputationMode(gcb,ComputationMode);
      settings: AttributesFormatString=%<BlockChoice>  OpenFcn=BringToFront(gcb);  MemberBlocks=Discrete-Time Integrator,Integrator
      settings: TemplateBlock=|
      | PreScanSimulinkLibrary/Configurable Subsystems/integral/Configurable
      | Subsystem1
  Configurable Subsystem3 : Subsystem  BlockChoice=Integrator  mask{ComputationMode=ComputationMode}
      mask prompts: ComputationMode "Computation mode:"
      mask init:
      | SetComputationMode(gcb,ComputationMode);
      settings: AttributesFormatString=%<BlockChoice>  OpenFcn=BringToFront(gcb);  MemberBlocks=Discrete-Time Integrator,Integrator
      settings: TemplateBlock=|
      | PreScanSimulinkLibrary/Configurable Subsystems/integral/Configurable
      | Subsystem1
  Configurable Subsystem4 : Subsystem  BlockChoice=Integrator  mask{ComputationMode=ComputationMode}
      mask prompts: ComputationMode "Computation mode:"
      mask init:
      | SetComputationMode(gcb,ComputationMode);
      settings: AttributesFormatString=%<BlockChoice>  OpenFcn=BringToFront(gcb);  MemberBlocks=Discrete-Time Integrator,Integrator
      settings: TemplateBlock=|
      | PreScanSimulinkLibrary/Configurable Subsystems/integral/Configurable
      | Subsystem1
  Configurable Subsystem5 : Subsystem  BlockChoice=Integrator  mask{ComputationMode=ComputationMode}
      mask prompts: ComputationMode "Computation mode:"
      mask init:
      | SetComputationMode(gcb,ComputationMode);
      settings: AttributesFormatString=%<BlockChoice>  OpenFcn=BringToFront(gcb);  MemberBlocks=Discrete-Time Integrator,Integrator
      settings: TemplateBlock=|
      | PreScanSimulinkLibrary/Configurable Subsystems/integral/Configurable
      | Subsystem1
  Configurable Subsystem9 : Subsystem  BlockChoice=Derivative  mask{ComputationMode=ComputationMode}
      mask prompts: ComputationMode "Computation mode:"
      mask init:
      | SetComputationMode(gcb,ComputationMode);
      settings: AttributesFormatString=%<BlockChoice>  OpenFcn=BringToFront(gcb);  MemberBlocks=Derivative,Discrete Derivative
      settings: TemplateBlock=|
      | PreScanSimulinkLibrary/Configurable Subsystems/Derivative/Configurable
      | Subsystem
  Constant : Constant  Value=p.g
  Constant1 : Constant  Value=p.VehMCSwitch
  D_roll : Fcn  Expr=u(1)*6*(p.df+p.dr)/2*p.width^2/2
  DampRateFront : Gain  Gain=p.df  SaturateOnIntegerOverflow=on  OutDataTypeStr=Inherit: Same as input  ParamDataTypeStr=Inherit: Same as input
  DampRateRear : Gain  Gain=p.dr  SaturateOnIntegerOverflow=on  OutDataTypeStr=Inherit: Same as input  ParamDataTypeStr=Inherit: Same as input
  Fcn : Fcn  Expr=u(1)-p.a*u(3)-u(5)
  Fcn1 : Fcn  Expr=u(2)-p.a*u(4)-u(6)
  Fcn2 : Fcn  Expr=u(2)+p.b*u(4)-u(8)
  Fcn3 : Fcn  Expr=u(1)+p.b*u(3)-u(7)
  Inertia : Gain  Gain=1/p.J_yy  SaturateOnIntegerOverflow=on  OutDataTypeStr=Inherit: Same as input  ParamDataTypeStr=Inherit: Same as input
  Inertia2 : Gain  Gain=p.m*p.hcog  SaturateOnIntegerOverflow=on  OutDataTypeStr=Inherit: Same as input  ParamDataTypeStr=Inherit: Same as input
  Jxx_roll = M*L^2 : Fcn  Expr=u(1)/(p.m*p.hcog^2)
  Mass : Gain  Gain=1/p.m  SaturateOnIntegerOverflow=on  OutDataTypeStr=Inherit: Same as input  ParamDataTypeStr=Inherit: Same as input
  Mass1 : Gain  Gain=p.m  SaturateOnIntegerOverflow=on  OutDataTypeStr=Inherit: Same as input  ParamDataTypeStr=Inherit: Same as input
  Multiport Switch : MultiPortSwitch  Inputs=2
  Multiport Switch1 : MultiPortSwitch  Inputs=2
  Mux : Mux  Inputs=8
  Mux1 : Mux  Inputs=2
  Product : Product  RndMeth=Zero
  Product1 : Product  RndMeth=Zero
  Product2 : Product  RndMeth=Zero
  SpringStiffnessFront : Gain  Gain=p.cf  SaturateOnIntegerOverflow=on  OutDataTypeStr=Inherit: Same as input  ParamDataTypeStr=Inherit: Same as input
  SpringStiffnessRear : Gain  Gain=p.cr  SaturateOnIntegerOverflow=on  OutDataTypeStr=Inherit: Same as input  ParamDataTypeStr=Inherit: Same as input
  Sum : Sum  Inputs=-+-  SaturateOnIntegerOverflow=on  InputSameDT=on  OutDataTypeStr=Inherit: Same as first input
  Sum1 : Sum  Inputs=--  SaturateOnIntegerOverflow=on  InputSameDT=on  OutDataTypeStr=Inherit: Same as first input
  Sum2 : Sum  Inputs=+--  SaturateOnIntegerOverflow=on  InputSameDT=on  OutDataTypeStr=Inherit: Same as first input
  Sum3 : Sum  Inputs=+++  SaturateOnIntegerOverflow=on  InputSameDT=on  OutDataTypeStr=Inherit: Same as first input
  Sum4 : Sum  SaturateOnIntegerOverflow=on  InputSameDT=on  OutDataTypeStr=Inherit: Same as first input
  Sum5 : Sum  SaturateOnIntegerOverflow=on  InputSameDT=on  OutDataTypeStr=Inherit: Same as first input
  Trigonometric Function : Trigonometry  Operator=cos
  Trigonometric Function1 : Trigonometry
  Trigonometric Function2 : Trigonometry  Operator=atan2
  Trigonometric Function3 : Trigonometry  Operator=cos
  due to sign convention : Gain  Gain=-1  SaturateOnIntegerOverflow=on  OutDataTypeStr=Inherit: Same as input  ParamDataTypeStr=Inherit: Same as input
  fcn : Fcn  Expr=u(1)*u(2)
  gain : Gain  Gain=p.a  SaturateOnIntegerOverflow=on  OutDataTypeStr=Inherit: Same as input  ParamDataTypeStr=Inherit: Same as input
  gain3 : Gain  Gain=p.b  SaturateOnIntegerOverflow=on  OutDataTypeStr=Inherit: Same as input  ParamDataTypeStr=Inherit: Same as input
  gravity : Constant  Value=p.g
  hcog : Gain  Gain=p.hcog  SaturateOnIntegerOverflow=on  OutDataTypeStr=Inherit: Same as input  ParamDataTypeStr=Inherit: Same as input
  pitchAngle_[rad] : Outport  VectorParamsAs1DForOutWhenUnconnected=off
  vz_[ms-1] : Outport  Port=2  VectorParamsAs1DForOutWhenUnconnected=off
  RollAngle_[rad] : Outport  Port=3  VectorParamsAs1DForOutWhenUnconnected=off
  RollRate_[rads-1] : Outport  Port=4  VectorParamsAs1DForOutWhenUnconnected=off
  wires:
  Sum3/1 -> Mass1/1  "sumForce_[N]"
  Sum1/1 -> Mass/1  "sumForce_[N]"
  Sum/1 -> Inertia/1  "sumTorque_[Nm]"
  Product2/1 -> Sum3/3
  Trigonometric Function3/1 -> Product2/2
  fcn/1 -> Product2/1
  dYaw/1 -> Mux1/2
  vx/1 -> Mux1/1
  Mux1/1 -> fcn/1
  Configurable Subsystem9/1(Out1) -> Multiport Switch1/3
  Multiport Switch1/1 -> RollRate_[rads-1]/1
  Multiport Switch/1 -> RollAngle_[rad]/1
  Constant1/1 -> Multiport Switch1/1, Multiport Switch/1
  gravity/1 -> Trigonometric Function2/2
  Trigonometric Function2/1 -> due to sign convention/1
  due to sign convention/1 -> Multiport Switch/3, Configurable Subsystem9/1(In1)
  Fcn2/1 -> DampRateRear/1
  Fcn3/1 -> SpringStiffnessRear/1
  Fcn1/1 -> DampRateFront/1
  Fcn/1 -> SpringStiffnessFront/1
  Mux/1 -> Fcn1/1, Fcn/1, Fcn3/1, Fcn2/1
  D_roll/1 -> Sum2/3
  C_roll/1 -> Sum2/2
  hcog/1 -> Sum2/1
  Mass1/1 -> hcog/1
  Product1/1 -> Sum3/2
  Product/1 -> Sum3/1
  Constant/1 -> Product1/2
  Trigonometric Function1/1 -> Product1/1
  ay/1 -> Trigonometric Function2/1, Product/1
  Trigonometric Function/1 -> Product/2
  Configurable Subsystem/1(Out1) -> Multiport Switch/2, Trigonometric Function3/1, Trigonometric Function/1, Trigonometric Function1/1, C_roll/1
  Configurable Subsystem5/1(Out1) -> Multiport Switch1/2, D_roll/1, Configurable Subsystem/1(In1)
  Jxx_roll = M*L^2/1 -> Configurable Subsystem5/1(In1)  "RollRate_[rads-2]"
  Sum2/1 -> Jxx_roll = M*L^2/1  "sumTorque_[N]"
  Sum5/1 -> Sum1/2, gain3/1
  Sum4/1 -> gain/1, Sum1/1
  Configurable Subsystem3/1(Out1) -> pitchAngle_[rad]/1, Mux/3  "PitchAngle_[rad]"
  gain/1 -> Sum/2
  gain3/1 -> Sum/3
  SpringStiffnessRear/1 -> Sum5/1  "FspringRear"
  DampRateRear/1 -> Sum5/2  "FdampRear"
  DampRateFront/1 -> Sum4/2  "FdampFront"
  SpringStiffnessFront/1 -> Sum4/1  "FspringFront"
  Configurable Subsystem4/1(Out1) -> Mux/1  "z_[m]"
  dzRear_[ms-1]/1 -> Mux/8
  zRear_[m]/1 -> Mux/7
  dzFront_[ms-1]/1 -> Mux/6
  zFront_[m]/1 -> Mux/5
  Inertia2/1 -> Sum/1
  ax/1 -> Inertia2/1
  Configurable Subsystem1/1(Out1) -> vz_[ms-1]/1, Mux/2, Configurable Subsystem4/1(In1)  "vz_[ms-1]"
  Mass/1 -> Configurable Subsystem1/1(In1)
  Configurable Subsystem2/1(Out1) -> Mux/4, Configurable Subsystem3/1(In1)  "dPitchAngle[rads-1]"
  Inertia/1 -> Configurable Subsystem2/1(In1)

== system Traffic_Light_cs/CAR_Main/Dynamics_Simple/Chassis/FrontTyre/AlphaFront ==
  In : Inport
  Abs : Abs
  Compare To Constant : simulink/Logic and Bit Operations/Compare To Constant  relop=>  const=0  OutDataTypeStr=uint8  ZeroCross=off
  Enabled Subsystem : Subsystem  TreatAsAtomicUnit=on
  Selector : Selector  IndexOptions=Index vector (dialog)  Indices=1  OutputSizes=1
  Alpha : Outport  VectorParamsAs1DForOutWhenUnconnected=off
  wires:
  Abs/1 -> Compare To Constant/1
  In/1 -> Selector/1, Enabled Subsystem/1(In)
  Enabled Subsystem/1(Alpha) -> Alpha/1
  Compare To Constant/1 -> Enabled Subsystem/Enable
  Selector/1 -> Abs/1

== system Traffic_Light_cs/CAR_Main/Dynamics_Simple/Chassis/FrontTyre/Configurable Subsystem ==
  In1 : Inport
  In2 : Inport  Port=2
  Integrator : Integrator  ExternalReset=level  LimitOutput=on  UpperSaturationLimit=1  LowerSaturationLimit=-1
  Out1 : Outport
  wires:
  In1/1 -> Integrator/1
  In2/1 -> Integrator/2
  Integrator/1 -> Out1/1

== system Traffic_Light_cs/CAR_Main/Dynamics_Simple/Chassis/FrontTyre/Configurable Subsystem1 ==
  In1 : Inport
  In2 : Inport  Port=2
  Integrator : Integrator  ExternalReset=level
  Out1 : Outport
  wires:
  In1/1 -> Integrator/1
  In2/1 -> Integrator/2
  Integrator/1 -> Out1/1

== system Traffic_Light_cs/CAR_Main/Dynamics_Simple/Chassis/FrontTyre/Prevent_instability_at_low_Vx ==
  note: |vx|
  alpha[rad] : Inport
  In : Inport  Port=2
  Divide : Product  Inputs=**
  Lookup Table : Lookup  InputValues="[0    2.5   ]"  Table="[0.01    1]"  LookUpMeth=Interpolation-Use End Values
  Selector : Selector  InputPortWidth=3  IndexOptions=Index vector (dialog)  Indices=[1]  OutputSizes=1
  alpha [rad] : Outport  VectorParamsAs1DForOutWhenUnconnected=off
  wires:
  Divide/1 -> alpha [rad]/1
  alpha[rad]/1 -> Divide/1
  Selector/1 -> Lookup Table/1
  Lookup Table/1 -> Divide/2
  In/1 -> Selector/1

== system Traffic_Light_cs/CAR_Main/Dynamics_Simple/Chassis/MuxDynState/Configurable Subsystem1 ==
  In1 : Inport
  Integrator : Integrator
  Out1 : Outport
  wires:
  In1/1 -> Integrator/1
  Integrator/1 -> Out1/1

== system Traffic_Light_cs/CAR_Main/Dynamics_Simple/Chassis/MuxDynState/Transformation_BODY2GLOBAL ==
  Vvector_BODY_[m/s] : Inport
  angles_BODYwrtGLOB_[rad] : Inport  Port=2
  Dot Product : DotProduct  InputSameDT=on  OutDataTypeStr=Inherit: Inherit via internal rule
  Dot Product1 : DotProduct  InputSameDT=on  OutDataTypeStr=Inherit: Inherit via internal rule
  Dot Product2 : DotProduct  InputSameDT=on  OutDataTypeStr=Inherit: Inherit via internal rule
  Fcn10 : Fcn  Expr=cos(u(1))*sin(u(2))*sin(u(3))-sin(u(1))*cos(u(3))
  Fcn11 : Fcn  Expr=cos(u(1))*sin(u(2))*cos(u(3))+sin(u(1))*sin(u(3))
  Fcn12 : Fcn  Expr=sin(u(1))*cos(u(2))
  Fcn13 : Fcn  Expr=sin(u(1))*sin(u(2))*sin(u(3))+cos(u(1))*cos(u(3))
  Fcn14 : Fcn  Expr=sin(u(1))*sin(u(2))*cos(u(3))-cos(u(1))*sin(u(3))
  Fcn15 : Fcn  Expr=-sin(u(2))
  Fcn16 : Fcn  Expr=cos(u(2))*sin(u(3))
  Fcn17 : Fcn  Expr=cos(u(2))*cos(u(3))
  Fcn9 : Fcn  Expr=cos(u(1))*cos(u(2))
  Mux1 : Mux  Inputs=9
  Mux3 : Mux  Inputs=3
  Selector : Selector  InputPortWidth=9  IndexOptions=Index vector (dialog)  Indices=[1 2 3]  OutputSizes=1
  Selector1 : Selector  InputPortWidth=9  IndexOptions=Index vector (dialog)  Indices=[4 5 6]  OutputSizes=1
  Selector2 : Selector  InputPortWidth=9  IndexOptions=Index vector (dialog)  Indices=[7 8 9]  OutputSizes=1
  rot_xyz 2 rot_zyx : Selector  InputPortWidth=3  IndexOptions=Index vector (dialog)  Indices=[3 2 1]  OutputSizes=1
  Vvector_GLOBAL_[m/s] : Outport  VectorParamsAs1DForOutWhenUnconnected=off
  wires:
  angles_BODYwrtGLOB_[rad]/1 -> rot_xyz 2 rot_zyx/1
  Mux3/1 -> Vvector_GLOBAL_[m/s]/1
  rot_xyz 2 rot_zyx/1 -> Fcn17/1, Fcn16/1, Fcn15/1, Fcn14/1, Fcn13/1, Fcn12/1, Fcn11/1, Fcn10/1, Fcn9/1
  Dot Product1/1 -> Mux3/2
  Dot Product2/1 -> Mux3/3
  Selector2/1 -> Dot Product2/2
  Selector1/1 -> Dot Product1/2
  Dot Product/1 -> Mux3/1
  Vvector_BODY_[m/s]/1 -> Dot Product/1, Dot Product1/1, Dot Product2/1
  Selector/1 -> Dot Product/2
  Mux1/1 -> Selector2/1, Selector1/1, Selector/1  "RotationMatrix Visu"
  Fcn17/1 -> Mux1/9
  Fcn16/1 -> Mux1/8
  Fcn15/1 -> Mux1/7
  Fcn14/1 -> Mux1/6
  Fcn13/1 -> Mux1/5
  Fcn12/1 -> Mux1/4
  Fcn11/1 -> Mux1/3
  Fcn10/1 -> Mux1/2
  Fcn9/1 -> Mux1/1

== system Traffic_Light_cs/CAR_Main/Dynamics_Simple/Chassis/RearTyre/AlphaRear ==
  In : Inport
  Abs : Abs
  Compare To Constant : simulink/Logic and Bit Operations/Compare To Constant  relop=>  const=0  OutDataTypeStr=uint8  ZeroCross=off
  Enabled Subsystem : Subsystem  TreatAsAtomicUnit=on
  Selector : Selector  IndexOptions=Index vector (dialog)  Indices=1  OutputSizes=1
  Alpha : Outport  VectorParamsAs1DForOutWhenUnconnected=off
  wires:
  Abs/1 -> Compare To Constant/1
  In/1 -> Selector/1, Enabled Subsystem/1(In)
  Enabled Subsystem/1(Alpha) -> Alpha/1
  Compare To Constant/1 -> Enabled Subsystem/Enable
  Selector/1 -> Abs/1

== system Traffic_Light_cs/CAR_Main/Dynamics_Simple/Chassis/RearTyre/Configurable Subsystem ==
  In1 : Inport
  In2 : Inport  Port=2
  Integrator : Integrator  ExternalReset=level
  Out1 : Outport
  wires:
  In1/1 -> Integrator/1
  In2/1 -> Integrator/2
  Integrator/1 -> Out1/1

== system Traffic_Light_cs/CAR_Main/Dynamics_Simple/Chassis/RearTyre/Configurable Subsystem1 ==
  In1 : Inport
  In2 : Inport  Port=2
  Integrator : Integrator  ExternalReset=level  LimitOutput=on  UpperSaturationLimit=1  LowerSaturationLimit=-1
  Out1 : Outport
  wires:
  In1/1 -> Integrator/1
  In2/1 -> Integrator/2
  Integrator/1 -> Out1/1

== system Traffic_Light_cs/CAR_Ahead/Trajectories/Traj2State1/Traj2State2/Traj2MuxState_Ext/demux ==
  traj : Inport
  Demux : Demux  Outputs=18
  x : Outport
  y : Outport  Port=2
  z : Outport  Port=3
  velx : Outport  Port=4
  vely : Outport  Port=5
  velz : Outport  Port=6
  R : Outport  Port=7
  P : Outport  Port=8
  Y : Outport  Port=9
  velR : Outport  Port=10
  velP : Outport  Port=11
  velY : Outport  Port=12
  accx : Outport  Port=13
  accy : Outport  Port=14
  accz : Outport  Port=15
  accR : Outport  Port=16
  accP : Outport  Port=17
  accY : Outport  Port=18
  wires:
  Demux/18 -> accY/1
  Demux/17 -> accP/1
  Demux/16 -> accR/1
  Demux/15 -> accz/1
  Demux/14 -> accy/1
  Demux/13 -> accx/1
  Demux/12 -> velY/1
  Demux/11 -> velP/1
  Demux/10 -> velR/1
  Demux/9 -> velz/1
  Demux/8 -> vely/1
  Demux/7 -> velx/1
  Demux/6 -> Y/1
  Demux/5 -> P/1
  traj/1 -> Demux/1
  Demux/4 -> R/1
  Demux/3 -> z/1
  Demux/2 -> y/1
  Demux/1 -> x/1

== system Traffic_Light_cs/CAR_Main/Dynamics_Simple/Chassis/Bicycle_model_[XYZ]/Y & Yaw_Motion/Configurable Subsystem ==
  In1 : Inport
  In2 : Inport  Port=2
  Integrator : Integrator  ExternalReset=level
  Out1 : Outport
  wires:
  In1/1 -> Integrator/1
  In2/1 -> Integrator/2
  Integrator/1 -> Out1/1

== system Traffic_Light_cs/CAR_Main/Dynamics_Simple/Chassis/Bicycle_model_[XYZ]/Y & Yaw_Motion/Configurable Subsystem1 ==
  In1 : Inport
  Integrator : Integrator
  Out1 : Outport
  wires:
  In1/1 -> Integrator/1
  Integrator/1 -> Out1/1

== system Traffic_Light_cs/CAR_Main/Dynamics_Simple/Chassis/Bicycle_model_[XYZ]/Y & Yaw_Motion/Configurable Subsystem2 ==
  In1 : Inport
  In2 : Inport  Port=2
  Integrator : Integrator  ExternalReset=level
  Out1 : Outport
  wires:
  In1/1 -> Integrator/1
  In2/1 -> Integrator/2
  Integrator/1 -> Out1/1

== system Traffic_Light_cs/CAR_Main/Dynamics_Simple/Chassis/Bicycle_model_[XYZ]/Z, Pitch_Motion & Roll_Motion/Configurable Subsystem ==
  In1 : Inport
  Integrator : Integrator  LimitOutput=on  UpperSaturationLimit=5*pi/180  LowerSaturationLimit=-5*pi/180
  Out1 : Outport
  wires:
  In1/1 -> Integrator/1
  Integrator/1 -> Out1/1

== system Traffic_Light_cs/CAR_Main/Dynamics_Simple/Chassis/Bicycle_model_[XYZ]/Z, Pitch_Motion & Roll_Motion/Configurable Subsystem1 ==
  In1 : Inport
  Integrator : Integrator
  Out1 : Outport
  wires:
  In1/1 -> Integrator/1
  Integrator/1 -> Out1/1

== system Traffic_Light_cs/CAR_Main/Dynamics_Simple/Chassis/Bicycle_model_[XYZ]/Z, Pitch_Motion & Roll_Motion/Configurable Subsystem2 ==
  In1 : Inport
  Integrator : Integrator
  Out1 : Outport
  wires:
  In1/1 -> Integrator/1
  Integrator/1 -> Out1/1

== system Traffic_Light_cs/CAR_Main/Dynamics_Simple/Chassis/Bicycle_model_[XYZ]/Z, Pitch_Motion & Roll_Motion/Configurable Subsystem3 ==
  In1 : Inport
  Integrator : Integrator
  Out1 : Outport
  wires:
  In1/1 -> Integrator/1
  Integrator/1 -> Out1/1

== system Traffic_Light_cs/CAR_Main/Dynamics_Simple/Chassis/Bicycle_model_[XYZ]/Z, Pitch_Motion & Roll_Motion/Configurable Subsystem4 ==
  In1 : Inport
  Integrator : Integrator
  Out1 : Outport
  wires:
  In1/1 -> Integrator/1
  Integrator/1 -> Out1/1

== system Traffic_Light_cs/CAR_Main/Dynamics_Simple/Chassis/Bicycle_model_[XYZ]/Z, Pitch_Motion & Roll_Motion/Configurable Subsystem5 ==
  In1 : Inport
  Integrator : Integrator
  Out1 : Outport
  wires:
  In1/1 -> Integrator/1
  Integrator/1 -> Out1/1

== system Traffic_Light_cs/CAR_Main/Dynamics_Simple/Chassis/Bicycle_model_[XYZ]/Z, Pitch_Motion & Roll_Motion/Configurable Subsystem9 ==
  In1 : Inport
  Derivative : Derivative
  Out1 : Outport
  wires:
  In1/1 -> Derivative/1
  Derivative/1 -> Out1/1

== system Traffic_Light_cs/CAR_Main/Dynamics_Simple/Chassis/FrontTyre/AlphaFront/Enabled Subsystem ==
  In : Inport
  Enable : EnablePort  PropagateVarSize=During execution
  AlphaFront : Fcn  Expr=-atan( (u(2)+u(3)*p.a)/u(1) )
  Alpha : Outport  OutputWhenDisabled=reset  InitialOutput=[0]  VectorParamsAs1DForOutWhenUnconnected=off
  wires:
  In/1 -> AlphaFront/1
  AlphaFront/1 -> Alpha/1

== system Traffic_Light_cs/CAR_Main/Dynamics_Simple/Chassis/RearTyre/AlphaRear/Enabled Subsystem ==
  In : Inport
  Enable : EnablePort  PropagateVarSize=During execution
  AlphaRear : Fcn  Expr=-atan( (u(2)-u(3)*p.b)/u(1) )
  Alpha : Outport  OutputWhenDisabled=reset  InitialOutput=[0]  VectorParamsAs1DForOutWhenUnconnected=off
  wires:
  In/1 -> AlphaRear/1
  AlphaRear/1 -> Alpha/1

== stateflow chart Traffic_Light_cs/CAR_Ahead/Decision/Chart ==
  state Initial_State
  state Decision_State
  (default) -> Initial_State
  Initial_State -> Decision_State : [Dis_Car2Light_0919_100<=500]{Decision_Call;}
  Decision_State -> Initial_State [order 2]
  Decision_State -> Initial_State [order 1] : [Dis_Car2Light_0919_100>500]
  data: Dis_Car2Light_0919_100 input
  events: Decision_Call output FUNCTION_CALL_EVENT

== stateflow chart Traffic_Light_cs/CAR_Ahead/Decision/Function-Call Subsystem/Chart ==
  state Initial
  state Camera
  (default) -> Initial
  Camera -> Initial
  Initial -> Camera : [Traffic_State<0]
      | {Camera_Call;
      | }
  data: Traffic_State input
  events: Camera_Call output FUNCTION_CALL_EVENT

== matlab function Traffic_Light_cs/CAR_Main/Decision/Function-Call Subsystem/Speed Decision by Q_leaning/MATLAB Function1 ==
  data: u1 input; a output; u2 input; u3 input; u4 input; u5 input
function a = a_cal(u1,u2,u3,u4,u5)
max=0;
s=0;
if u1>max
    max = u1;
    s=-1.2;
end
if u2>max
    max = u2;
    s=-0.4;
end
if u3>max
    max = u3;
    s=0;
end
if u4>max
    max = u4;
    s=0.4;
end
if u5>max
    max = u5;
    s=1.2;
end
a=s;

== stateflow chart Traffic_Light_cs/CAR_Ahead/Decision/Function-Call Subsystem/Subsystem/Delay ==
  state Initial
    en:
    Local_State=Light_State_0919_100;
    count1=500;
  state Delay
    en:
    Light_State_End=Local_State;
  (default) -> Initial
  Initial -> Delay : [count1>0]
  Delay -> Initial [order 1] : [count1<=0]
  Delay -> Delay [order 3] : [Local_State~=Light_State_0919_100&&Light_State_0919_100==-1]
      | {count1=count1-1;}
  Delay -> Delay [order 2] : [Local_State~=Light_State_0919_100&&Light_State_0919_100>=0]
      | {count1=0;}
  data: Light_State_0919_100 input; Light_State_End output; Local_State local; count1 local
